simulink model "mpc_prueba_raul"  (R2017a)
settings: Solver=VariableStepAuto  StartTime=0.0  StopTime=10.0  MaxStep=1e-4  RelTol=1e-3
values from neighbouring files (symbols this model uses):
  Ap = [-1/(R*C)   1/C        0    -1/C      1/C        0 ... (first row only)    [GeneradoresInterconectados.m]
  Bp = [    0      0 ... (first row only)    [GeneradoresInterconectados.m]
  Cp = [    1      0 ... (first row only)    [GeneradoresInterconectados.m]
  Dp = zeros(2,2)    [GeneradoresInterconectados.m]
  I2 = 18    [GeneradoresInterconectados.m]
  Vabc = 160    [GeneradoresInterconectados.m]
libraries: mpclib x1, powerlib x1
settings Model: Creator=Administrador  LastModifiedBy=Administrador

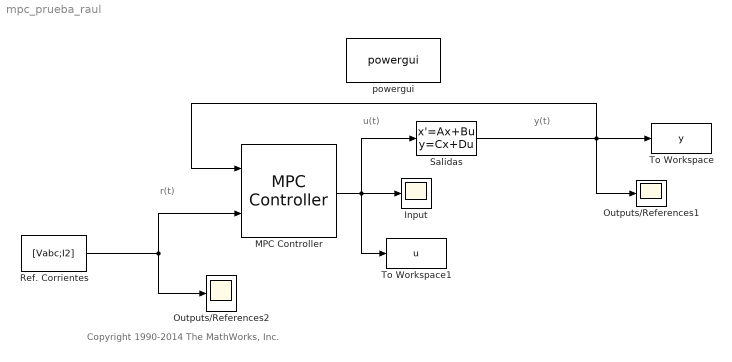
== system mpc_prueba_raul ==
  note: y(t)
  note: r(t)
  note: u(t)
  note: Copyright 1990-2014 The MathWorks, Inc.
  Input : Scope
  MPC Controller : mpclib/MPC Controller  mpcobj=mpcobj  x0=[]  is_multiple=0  enable_value=0  return_u0=off  ref_from_ws=off  ref_signal_name=[]  ref_preview=on  md_from_ws=off  md_signal_name=[]  md_preview=on  from_project=off  project_file=MPCtask.mat  md_inport=off  mv_inport=off  cost_outport=off  return_sequence=off  return_qpstatus=off  return_state=off  state_inport=off  lims_inport=off  ywt_inport=off  is_designfromscratch=0  uwt_inport=off  duwt_inport=off  rhoeps_inport=off  uref_inport=off  n_ts=0.1  n_mv=2  n_md=0  n_ud=0  n_mo=2  n_uo=0  BlockDataType=double  SampleTimeInherited=off  switch_inport=off
  Outputs/References1 : Scope
  Outputs/References2 : Scope
  Ref. Corrientes : Constant  Value=[Vabc;I2]
  Salidas : StateSpace  A=Ap  B=Bp  C=Cp  D=Dp  X0=0
  To Workspace : ToWorkspace  VariableName=y  SampleTime=-1
      settings: MaxDataPoints=Inf
  To Workspace1 : ToWorkspace  VariableName=u  SampleTime=-1
      settings: MaxDataPoints=Inf
  powergui : powerlib/powergui  SimulationMode=Continuous  SampleTime=50e-6  frequency=60  Iterations=50  frequencyindice=0  Pbase=100e6  ErrMax=1e-4  UnitsV=kV  UnitsW=MW  buscounter=0  FunctionMessages=off  echomessages=off  EnableUseOfTLC=off  CurrentSourceSwitches=off  DisableSnubberDevices=off  DisableRonSwitches=off  DisableVfSwitches=off  DisplayEquations=off  SolverType=Tustin/Backward Euler (TBE)  Interpol=off  ExternalGateDelay=off  methode=off  Ts=100  x0status=blocks  SPID=on  SwTol=0  HookPort=off  RestoreLinks=warning  ResistiveCurrentMeasurement=off  Frange=[0:2:500]  Ylog=off  Xlog=on  ShowGrid=off  save=off  variable=ZData  structure=sps1phPWM1_str  ZoomFFT=on  StartTime=0.1-2/60  cycles=2  DisplayStyle=1  fundamental=60  FreqAxis=off  MaxFrequency=5000  frequencyindicesteady=1  RmsSteady=1  display=off
  wires:
  Salidas/1 -> To Workspace/1, Outputs/References1/1, MPC Controller/1
  Ref. Corrientes/1 -> MPC Controller/2, Outputs/References2/1
  MPC Controller/1 -> Salidas/1, Input/1, To Workspace1/1
